simulink library "sm_visualization"  (R2016b)
settings: Solver=VariableStepAuto  StartTime=0.0  StopTime=10.0  RelTol=1e-3
undefined symbols (not defined in the file or in its folder): fsw_params
libraries: aerolibutil x2, dspmathops x2, sm_animate_cubesat_lib x1
settings Model: Creator=Taylor  LastModifiedBy=Taylor

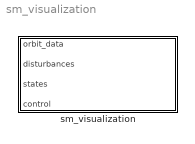
== system sm_visualization ==
  sm_visualization : Subsystem

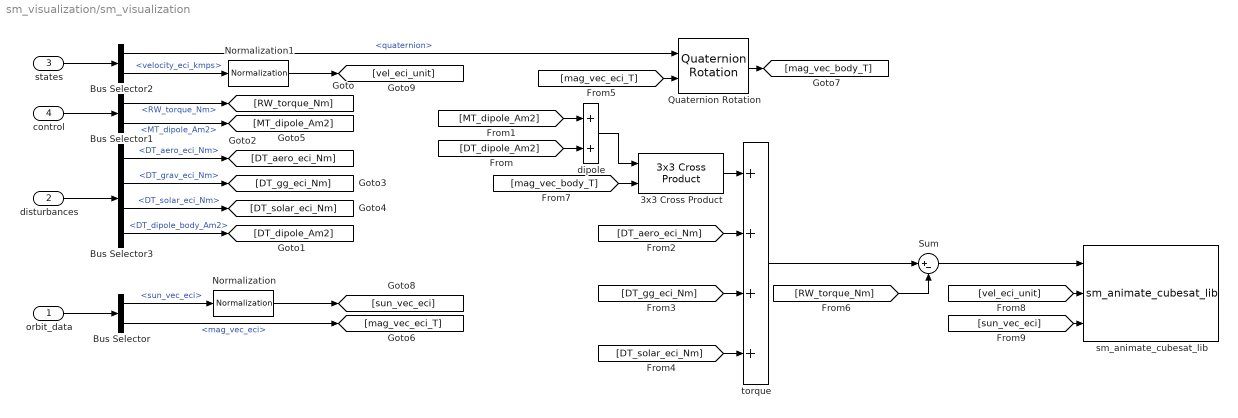
== system sm_visualization/sm_visualization ==
  orbit_data : Inport  OutDataTypeStr=Bus: orbit_data
  disturbances : Inport  Port=2  OutDataTypeStr=Bus: disturbances
  states : Inport  Port=3  OutDataTypeStr=Bus: states
  control : Inport  Port=4  OutDataTypeStr=Bus: control
  3x3 Cross Product : aerolibutil/3x3 Cross Product
  Bus Selector : BusSelector  OutputSignals=sun_vec_eci,mag_vec_eci
  Bus Selector1 : BusSelector  OutputSignals=RW_torque_Nm,MT_dipole_Am2
  Bus Selector2 : BusSelector  OutputSignals=quaternion,velocity_eci_kmps
  Bus Selector3 : BusSelector  OutputSignals=DT_aero_eci_Nm,DT_grav_eci_Nm,DT_solar_eci_Nm,DT_dipole_body_Am2
  Normalization : dspmathops/Normalization  NormType=2-norm  Bias=1e-10  NormOver=Each column  Dimension=1  outputDataTypeStr=Inherit: Same as product output  outputLastDataTypeStr=Inherit: Same as product output  outputMin=[]  outputMax=[]  accumDataTypeStr=Inherit: Same as product output  accumLastDataTypeStr=Inherit: Same as product output  roundingMode=Floor  overflowMode=off
  Normalization1 : dspmathops/Normalization  NormType=2-norm  Bias=1e-10  NormOver=Each column  Dimension=1  outputDataTypeStr=Inherit: Same as product output  outputLastDataTypeStr=Inherit: Same as product output  outputMin=[]  outputMax=[]  accumDataTypeStr=Inherit: Same as product output  accumLastDataTypeStr=Inherit: Same as product output  roundingMode=Floor  overflowMode=off
  Quaternion Rotation : aerolibutil/Quaternion Rotation
  Sum : Sum  Inputs=|+-
  dipole : Sum  Inputs=2
  sm_animate_cubesat_lib : sm_animate_cubesat_lib/sm_animate_cubesat_lib  L=fsw_params.bus.dx  W=fsw_params.bus.dy  H=fsw_params.bus.dz  Mass=fsw_params.bus.mass  CoM=fsw_params.bus.CoM  moment_inertia=diag(fsw_params.bus.inertia)  prod_inertia=fsw_params.bus.prod_inertia
  torque : Sum  Inputs=4
  wires:
  orbit_data/1 -> Bus Selector/1
  Bus Selector/1 -> Normalization/1  "<sun_vec_eci>"
  control/1 -> Bus Selector1/1
  states/1 -> Bus Selector2/1
  disturbances/1 -> Bus Selector3/1
  Bus Selector2/2 -> Normalization1/1  "<velocity_eci_kmps>"
  [DT_gg_eci_Nm] -> torque/3
  [DT_aero_eci_Nm] -> torque/2
  3x3 Cross Product/1 -> torque/1
  [DT_solar_eci_Nm] -> torque/4
  Bus Selector3/4 -> [DT_dipole_Am2]  "<DT_dipole_body_Am2>"
  Bus Selector3/3 -> [DT_solar_eci_Nm]  "<DT_solar_eci_Nm>"
  Bus Selector3/2 -> [DT_gg_eci_Nm]  "<DT_grav_eci_Nm>"
  Bus Selector3/1 -> [DT_aero_eci_Nm]  "<DT_aero_eci_Nm>"
  [mag_vec_body_T] -> 3x3 Cross Product/2
  [MT_dipole_Am2] -> dipole/1
  [DT_dipole_Am2] -> dipole/2
  dipole/1 -> 3x3 Cross Product/1
  torque/1 -> Sum/1
  Bus Selector1/1 -> [RW_torque_Nm]  "<RW_torque_Nm>"
  Bus Selector1/2 -> [MT_dipole_Am2]  "<MT_dipole_Am2>"
  Quaternion Rotation/1 -> [mag_vec_body_T]
  Bus Selector2/1 -> Quaternion Rotation/1  "<quaternion>"
  Bus Selector/2 -> [mag_vec_eci_T]  "<mag_vec_eci>"
  [mag_vec_eci_T] -> Quaternion Rotation/2
  [RW_torque_Nm] -> Sum/2
  Sum/1 -> sm_animate_cubesat_lib/1
  Normalization/1 -> [sun_vec_eci]
  Normalization1/1 -> [vel_eci_unit]
  [vel_eci_unit] -> sm_animate_cubesat_lib/2
  [sun_vec_eci] -> sm_animate_cubesat_lib/3
